simulink model "Modele_pendule_c"  (R2020b)
settings: Solver=VariableStepAuto  StartTime=0.0  StopTime=20  RelTol=1e-3
undefined symbols (not defined in the file or in its folder): A, B, Kx
settings Model: Creator=georgesghazi  LastModifiedBy=georgesghazi

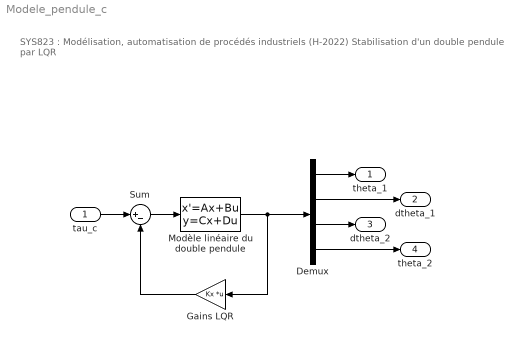
== system Modele_pendule_c ==
  note: SYS823 : Modélisation, automatisation de procédés industriels (H-2022)
      |
      | Stabilisation d'un double pendule par LQR
  tau_c : Inport
  Demux : Demux
  Gains LQR : Gain  Gain=Kx  Multiplication=Matrix(K*u) (u vector)
  Modèle linéaire du double pendule : StateSpace  A=A  B=B  C=eye(4)  D=zeros(4, 1)  InitialCondition=0
  Sum : Sum  Inputs=|+-
  theta_1 : Outport
  dtheta_1 : Outport  Port=2
  dtheta_2 : Outport  Port=3
  theta_2 : Outport  Port=4
  wires:
  tau_c/1 -> Sum/1
  Sum/1 -> Modèle linéaire du double pendule/1
  Gains LQR/1 -> Sum/2
  Demux/1 -> theta_1/1
  Demux/3 -> dtheta_2/1
  Demux/2 -> dtheta_1/1
  Demux/4 -> theta_2/1
  Modèle linéaire du double pendule/1 -> Gains LQR/1, Demux/1
